simulink model "boilerplate"  (R2017b)
settings: Solver=VariableStepAuto  StartTime=0.0  StopTime=10.0  RelTol=1e-3
libraries: simulink x2, vrlib x2
settings Model: Creator=kenny.nguyen  LastModifiedBy=kenny.nguyen

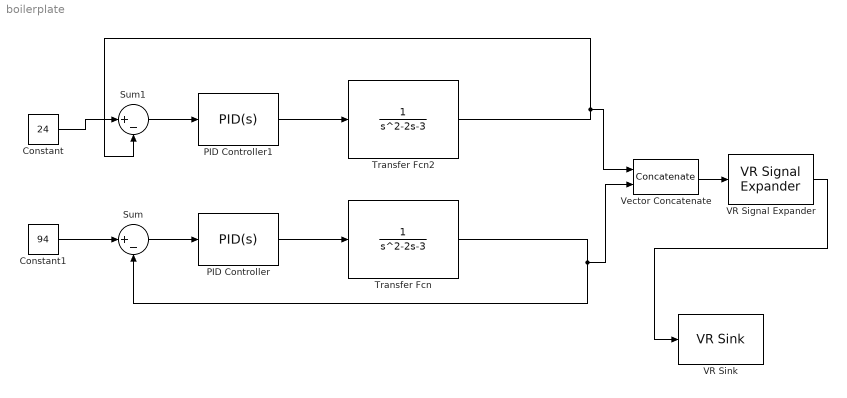
== system boilerplate ==
  Constant : Constant  Value=24
  Constant1 : Constant  Value=94
  PID Controller : simulink/Continuous/PID Controller  Controller=PID  TimeDomain=Continuous-time  SampleTime=-1  IntegratorMethod=Forward Euler  FilterMethod=Forward Euler  Form=Parallel  UseFilter=on  ControllerParametersSource=internal  P=31.4567913744569  I=18.637367158971  D=11.0760741229445  N=1241.76810994334  InitialConditionSource=internal  InitialConditionForIntegrator=0  InitialConditionForFilter=0  ExternalReset=none  LimitOutput=on  UpperSaturationLimit=inf  LowerSaturationLimit=-inf  LinearizeAsGain=on  AntiWindupMode=none  Kb=1  TrackingMode=off  Kt=1  PParamMin=0  PParamMax=100  IParamMin=0  IParamMax=100  DParamMin=0  DParamMax=100  NParamMin=[]  NParamMax=[]  KbParamMin=[]  KbParamMax=[]  KtParamMin=[]  KtParamMax=[]  POutMin=2  POutMax=2  POutDataTypeStr=double  PGainOutDataTypeStr=double  PProdOutDataTypeStr=double  IOutMin=2  IOutMax=2  IOutDataTypeStr=double  IGainOutDataTypeStr=double  IProdOutDataTypeStr=double  DOutMin=2  DOutMax=2  DOutDataTypeStr=double  DGainOutDataTypeStr=double  DProdOutDataTypeStr=double  NOutMin=2  NOutMax=2  NOutDataTypeStr=double  NGainOutDataTypeStr=double  NProdOutDataTypeStr=double  KbOutMin=[]  KbOutMax=[]  KtOutMin=[]  KtOutMax=[]  IntegratorOutMin=[]  IntegratorOutMax=[]  FilterOutMin=[]  FilterOutMax=[]  SumOutMin=[]  SumOutMax=[]  SumI1OutMin=[]  SumI1OutMax=[]  SumI2OutMin=[]  SumI2OutMax=[]  SumI3OutMin=[]  SumI3OutMax=[]  SumDOutMin=[]  SumDOutMax=[]  SaturationOutMin=[]  SaturationOutMax=[]  IntegratorContinuousStateAttributes=''  IntegratorStateMustResolveToSignalObject=off  IntegratorRTWStateStorageClass=Auto  FilterContinuousStateAttributes=''  FilterStateMustResolveToSignalObject=off  FilterRTWStateStorageClass=Auto  DifferentiatorICPrevScaledInput=0  DifferentiatorOutMin=[]  DifferentiatorOutMax=[]  InitialConditionSetting=State (most efficient)  FilterDiffOutCoefMin=[]  FilterDiffOutCoefMax=[]  SumDenOutMin=[]  SumDenOutMax=[]  SumNumOutMin=[]  SumNumOutMax=[]  ReciprocalOutMin=[]  ReciprocalOutMax=[]  DivideOutMin=[]  DivideOutMax=[]  TunerSelectOption=Transfer Function Based (PID Tuner App)
  PID Controller1 : simulink/Continuous/PID Controller  Controller=PID  TimeDomain=Continuous-time  SampleTime=-1  IntegratorMethod=Forward Euler  FilterMethod=Forward Euler  Form=Parallel  UseFilter=on  ControllerParametersSource=internal  P=19.9647149440043  I=10.3556779822916  D=8.62853293422472  N=941.977441589389  InitialConditionSource=internal  InitialConditionForIntegrator=0  InitialConditionForFilter=0  ExternalReset=none  LimitOutput=on  UpperSaturationLimit=inf  LowerSaturationLimit=-inf  LinearizeAsGain=on  AntiWindupMode=none  Kb=1  TrackingMode=off  Kt=1  PParamMin=0  PParamMax=100  IParamMin=0  IParamMax=100  DParamMin=0  DParamMax=100  NParamMin=[]  NParamMax=[]  KbParamMin=[]  KbParamMax=[]  KtParamMin=[]  KtParamMax=[]  POutMin=2  POutMax=2  POutDataTypeStr=double  PGainOutDataTypeStr=double  PProdOutDataTypeStr=double  IOutMin=2  IOutMax=2  IOutDataTypeStr=double  IGainOutDataTypeStr=double  IProdOutDataTypeStr=double  DOutMin=2  DOutMax=2  DOutDataTypeStr=double  DGainOutDataTypeStr=double  DProdOutDataTypeStr=double  NOutMin=2  NOutMax=2  NOutDataTypeStr=double  NGainOutDataTypeStr=double  NProdOutDataTypeStr=double  KbOutMin=[]  KbOutMax=[]  KtOutMin=[]  KtOutMax=[]  IntegratorOutMin=[]  IntegratorOutMax=[]  FilterOutMin=[]  FilterOutMax=[]  SumOutMin=[]  SumOutMax=[]  SumI1OutMin=[]  SumI1OutMax=[]  SumI2OutMin=[]  SumI2OutMax=[]  SumI3OutMin=[]  SumI3OutMax=[]  SumDOutMin=[]  SumDOutMax=[]  SaturationOutMin=[]  SaturationOutMax=[]  IntegratorContinuousStateAttributes=''  IntegratorStateMustResolveToSignalObject=off  IntegratorRTWStateStorageClass=Auto  FilterContinuousStateAttributes=''  FilterStateMustResolveToSignalObject=off  FilterRTWStateStorageClass=Auto  DifferentiatorICPrevScaledInput=0  DifferentiatorOutMin=[]  DifferentiatorOutMax=[]  InitialConditionSetting=State (most efficient)  FilterDiffOutCoefMin=[]  FilterDiffOutCoefMax=[]  SumDenOutMin=[]  SumDenOutMax=[]  SumNumOutMin=[]  SumNumOutMax=[]  ReciprocalOutMin=[]  ReciprocalOutMax=[]  DivideOutMin=[]  DivideOutMax=[]  TunerSelectOption=Transfer Function Based (PID Tuner App)
  Sum : Sum  Inputs=|+-  OutMin=2  OutMax=2
  Sum1 : Sum  Inputs=|+-  OutMin=2  OutMax=2
  Transfer Fcn : TransferFcn  Denominator=[1 -2 -3]
  Transfer Fcn2 : TransferFcn  Denominator=[1 -2 -3]
  VR Signal Expander : vrlib/VR Signal Expander  outwidth=4  outidx=[3 4]
      settings: SourceProductName=Simulink 3D Animation  SourceProductBaseCode=VR
  VR Sink : vrlib/VR Sink  InstantiateOnLoad=on  SampleTime=0.1  ViewEnable=on  RemoteChange=off  RemoteView=off  FieldsWritten=Axis.rotation.4.1.1.double  WorldFileName=telescope.wrl  WorldDescription=telescope  AutoView=on  VideoDimensions=[]  AllowVariableSize=off  FigureProperties="{'Position', 'Name', 'Viewpoint', 'CameraBound', 'CameraDirection', 'CameraPosition', 'CameraUpVector', 'ZoomFactor', 'Antialiasing', 'Headlight', 'Lighting', 'NavPanel', 'Sound', 'StatusBar', 'Stereo3D', 'Stereo3DCameraOffset', 'Stereo3DHIT', 'ToolBar', 'Textures', 'Transparency', 'Triad', 'Wireframe', 'NavZones', 'NavMode', 'NavSpeed', 'CaptureFileFormat', 'CaptureFileName', 'Record2DCompressMethod', 'Record2DCompressQuality', 'Record2D', 'Record2DFileName', 'Record2DFPS'; [5.0000000000000000e+00   9.2333333333333371e+01   5.7600000000000000e+02   3.5000000000000000e+02], 'telescope', '', 'on', [4.6342956941106372e-01   2.4051339830436472e-01  -8.5286947385374701e-01], [-3.3906517065484882e+00  -1.6694859278629286e+00   1.2684529366945936e+01], [-5.9947073307648091e-02   9.6876570506462012e-01   2.4062285239041259e-01], [1.0000000000000000e+00], 'on', 'on', 'on', 'halfbar', 'on', 'on', 'off', [1.0000000149011612e-01], [0.0000000000000000e+00], 'on', 'on', 'on', 'none', 'off', 'off', 'fly', 'normal', 'tif', '%f_anim_%n.tif', 'auto', [7.5000000000000000e+01], 'off', '%f_anim_%n.avi', 'auto'}"
      settings: SourceProductBaseCode=VR
  Vector Concatenate : Concatenate
  wires:
  Sum1/1 -> PID Controller1/1
  Constant1/1 -> Sum/1
  PID Controller1/1 -> Transfer Fcn2/1
  PID Controller/1 -> Transfer Fcn/1
  Sum/1 -> PID Controller/1
  Transfer Fcn2/1 -> Vector Concatenate/1, Sum1/2
  Transfer Fcn/1 -> Vector Concatenate/2, Sum/2
  Constant/1 -> Sum1/1
  Vector Concatenate/1 -> VR Signal Expander/1
  VR Signal Expander/1 -> VR Sink/1
